simulink model "Pendulum"  (R2021a)
settings: Solver=VariableStepAuto  StartTime=0.0  StopTime=80  RelTol=1e-3
undefined symbols (not defined in the file): c, d, g, J, L, m
libraries: simulink_extras x4, fuzblock x2
settings Model: Creator=ejbejaranos  LastModifiedBy=ejbejaranos

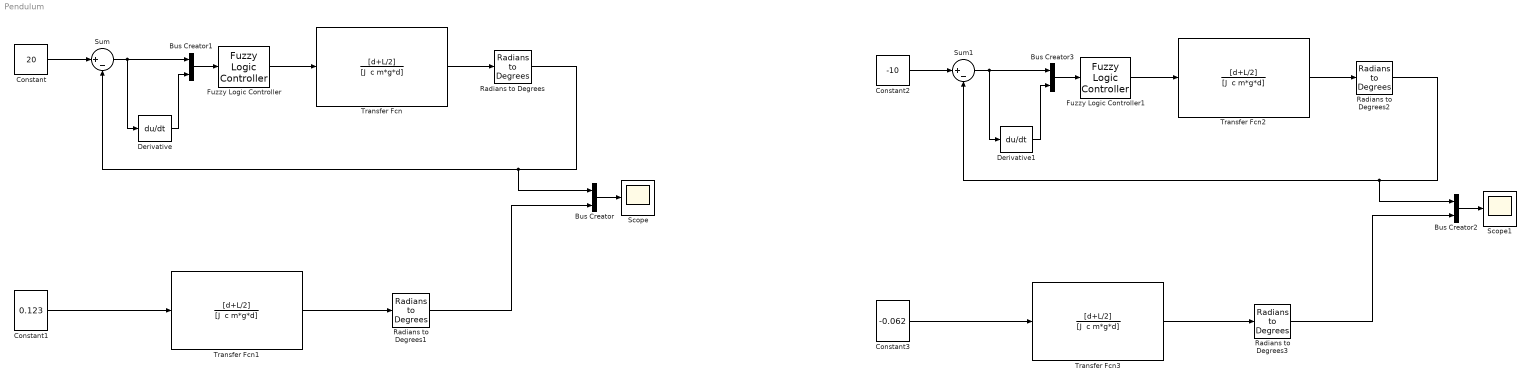
== system Pendulum ==
  Bus Creator{,1..3} (4 alike) : BusCreator  Inputs=2
  Constant : Constant  Value=20
  Constant1 : Constant  Value=0.123
  Constant2 : Constant  Value=-10
  Constant3 : Constant  Value=-0.062
  Derivative : Derivative
  Derivative1 : Derivative
  Fuzzy Logic Controller : fuzblock/Fuzzy Logic  Controller  FIS=Mandami  OutputSampleNumber=101  DataType=double  FuzzifiedInputs=off  RuleFiringStrengths=off  RuleOutputs=off  AggregatedOutputs=off  SimulateUsing=Interpreted execution  OutOfRangeInputValueMessage=warning  NoRuleFiredMessage=warning  EmptyOutputFuzzySetMessage=warning
  Fuzzy Logic Controller1 : fuzblock/Fuzzy Logic  Controller  FIS=Mandami  OutputSampleNumber=101  DataType=double  FuzzifiedInputs=off  RuleFiringStrengths=off  RuleOutputs=off  AggregatedOutputs=off  SimulateUsing=Interpreted execution  OutOfRangeInputValueMessage=warning  NoRuleFiredMessage=warning  EmptyOutputFuzzySetMessage=warning
  Radians to Degrees{,1..3} (4 alike) : simulink_extras/Transformations/Radians to Degrees
  Scope : Scope
  Scope1 : Scope
  Sum : Sum  Inputs=|+-
  Sum1 : Sum  Inputs=|+-
  Transfer Fcn{,1..3} (4 alike) : TransferFcn  Numerator=[d+L/2]  Denominator="[J  c m*g*d]"
  wires:
  Bus Creator/1 -> Scope/1
  Bus Creator1/1 -> Fuzzy Logic Controller/1
  Constant/1 -> Sum/1
  Sum/1 -> Derivative/1, Bus Creator1/1
  Derivative/1 -> Bus Creator1/2
  Fuzzy Logic Controller/1 -> Transfer Fcn/1
  Transfer Fcn/1 -> Radians to Degrees/1
  Radians to Degrees/1 -> Bus Creator/1, Sum/2
  Constant1/1 -> Transfer Fcn1/1
  Transfer Fcn1/1 -> Radians to Degrees1/1
  Radians to Degrees1/1 -> Bus Creator/2
  Constant3/1 -> Transfer Fcn3/1
  Radians to Degrees3/1 -> Bus Creator2/2
  Constant2/1 -> Sum1/1
  Fuzzy Logic Controller1/1 -> Transfer Fcn2/1
  Transfer Fcn3/1 -> Radians to Degrees3/1
  Bus Creator3/1 -> Fuzzy Logic Controller1/1
  Radians to Degrees2/1 -> Bus Creator2/1, Sum1/2
  Bus Creator2/1 -> Scope1/1
  Transfer Fcn2/1 -> Radians to Degrees2/1
  Derivative1/1 -> Bus Creator3/2
  Sum1/1 -> Derivative1/1, Bus Creator3/1
